simulink model "sol_mdl"  (R2024b)
settings: Solver=ode4  StartTime=0.0  StopTime=tf_sim  FixedStep=dt  RelTol=1e-3
values from neighbouring files (symbols this model uses):
  controller_coeffs = [Kp;Kd]    [init.m]
  q0_c1 = angle2quat(teta0_c1(3),teta0_c1(2),teta0_c1(1),'ZYX')    [init.m]
  q0_c2 = angle2quat(teta0_c2(3),teta0_c2(2),teta0_c2(1),'ZYX')    [init.m]
  qd_c1 = angle2quat(tetad_c1(3),tetad_c1(2),tetad_c1(1),'ZYX')    [init.m]
  qd_c2 = angle2quat(tetad_c2(3),tetad_c2(2),tetad_c2(1),'ZYX')    [init.m]
  so_c1 = Cbo'*sb0    [init.m]
  so_c2 = Cbo'*sb0    [init.m]
  system_parameters = [a; l; b; As; sigma; ms; mp; mr; mt; P]    [init.m]
  tetad_c2 = deg2rad([0 20 20]')    [init.m]
  w0_c1 = [0 5 5]'*1e-4    [init.m]
  w0_c2 = [0 0 0]'    [init.m]
libraries: aerolibutil x4, sharedtransform x2, simulink_extras x2
settings Model: Creator=Monster  LastModifiedBy=Monster

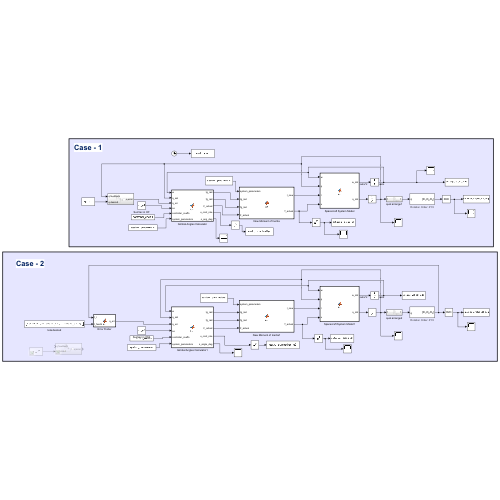
[thumbnail: Simulink's stored preview of the top-level diagram]
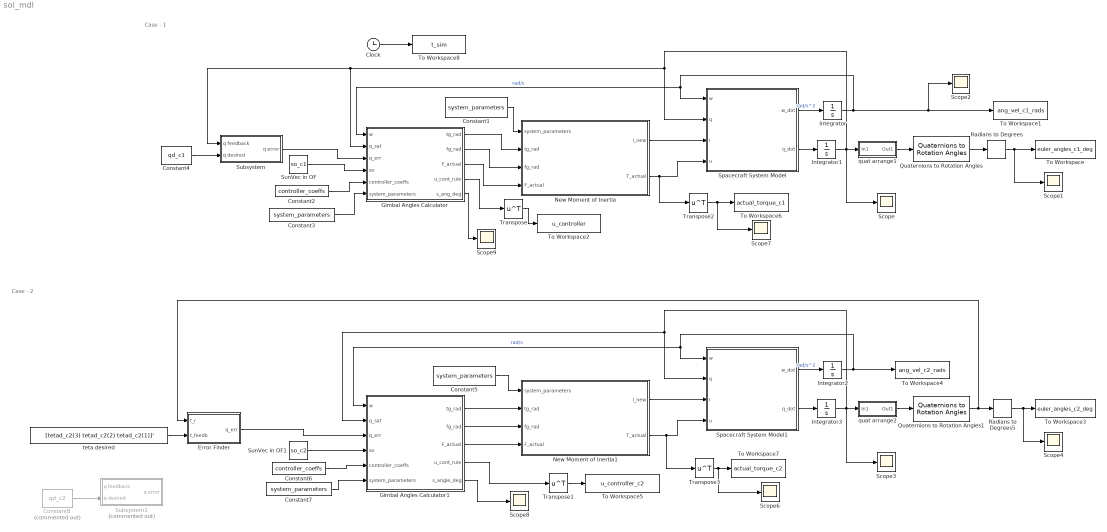
== system sol_mdl ==
  note: Case - 1
  note: Case - 2
  Clock : Clock
  Constant{1,3,5,7} (4 alike) : Constant  Value=system_parameters
  Constant2 : Constant  Value=controller_coeffs
  Constant4 : Constant  Value=qd_c1
  Constant6 : Constant  Value=controller_coeffs
  Constant8 : Constant  Commented=on  Value=qd_c2
  Error Finder : MATLAB Function  TreatAsAtomicUnit=on
  Gimbal Angles Calculator : MATLAB Function  TreatAsAtomicUnit=on
  Gimbal Angles Calculator1 : MATLAB Function  TreatAsAtomicUnit=on
  Integrator : Integrator  InitialCondition=w0_c1
  Integrator1 : Integrator  InitialCondition=[q0_c1(2:4)';q0_c1(1)]
  Integrator2 : Integrator  InitialCondition=w0_c2
  Integrator3 : Integrator  InitialCondition=[q0_c2(2:4)';q0_c2(1)]
  New Moment of Inertia : MATLAB Function  TreatAsAtomicUnit=on
  New Moment of Inertia1 : MATLAB Function  TreatAsAtomicUnit=on
  Quaternions to Rotation Angles : sharedtransform/Quaternions to Rotation Angles  rotationOrder=ZYX  aMode=aMode
  Quaternions to Rotation Angles1 : sharedtransform/Quaternions to Rotation Angles  rotationOrder=ZYX  aMode=aMode
  Radians to Degrees : simulink_extras/Transformations/Radians to Degrees
  Radians to Degrees5 : simulink_extras/Transformations/Radians to Degrees
  Scope{,1..4,6..9} (9 alike) : Scope
  Spacecraft System Model : MATLAB Function  TreatAsAtomicUnit=on
  Spacecraft System Model1 : MATLAB Function  TreatAsAtomicUnit=on
  Subsystem : Subsystem
  Subsystem1 : Subsystem  Commented=on
  SunVec in OF : Constant  Value=so_c1
  SunVec in OF1 : Constant  Value=so_c2
  To Workspace : ToWorkspace  VariableName=euler_angles_c1_deg  SampleTime=-1
      settings: Save2DSignal=2-D array (concatenate along first dimension)
  To Workspace1 : ToWorkspace  VariableName=ang_vel_c1_rads  SampleTime=-1
      settings: Save2DSignal=2-D array (concatenate along first dimension)
  To Workspace2 : ToWorkspace  VariableName=u_controller  SampleTime=-1
      settings: Save2DSignal=2-D array (concatenate along first dimension)
  To Workspace3 : ToWorkspace  VariableName=euler_angles_c2_deg  SampleTime=-1
      settings: Save2DSignal=2-D array (concatenate along first dimension)
  To Workspace4 : ToWorkspace  VariableName=ang_vel_c2_rads  SampleTime=-1
      settings: Save2DSignal=2-D array (concatenate along first dimension)
  To Workspace5 : ToWorkspace  VariableName=u_controller_c2  SampleTime=-1
      settings: Save2DSignal=2-D array (concatenate along first dimension)
  To Workspace6 : ToWorkspace  VariableName=actual_torque_c1  SampleTime=-1
      settings: Save2DSignal=2-D array (concatenate along first dimension)
  To Workspace7 : ToWorkspace  VariableName=actual_torque_c2  SampleTime=-1
      settings: Save2DSignal=2-D array (concatenate along first dimension)
  To Workspace8 : ToWorkspace  VariableName=t_sim  SampleTime=-1
      settings: Save2DSignal=2-D array (concatenate along first dimension)
  Transpose{,1..3} (4 alike) : Math  Operator=transpose
  quat arrange1 : Subsystem
  quat arrange2 : Subsystem
  teta desired : Constant  Value=[tetad_c2(3) tetad_c2(2) tetad_c2(1)]'
  wires:
  Spacecraft System Model/2(q_dot) -> Integrator1/1
  Spacecraft System Model/1(w_dot) -> Integrator/1  "rad/s^2"
  Integrator/1 -> Scope2/1, To Workspace1/1, Gimbal Angles Calculator/1(w), Spacecraft System Model/1(w)  "rad/s"
  Constant1/1 -> New Moment of Inertia/1(system_parameters)
  New Moment of Inertia/1(I_new) -> Spacecraft System Model/3(I)
  Quaternions to Rotation Angles/1 -> Radians to Degrees/1
  Constant2/1 -> Gimbal Angles Calculator/5(controller_coeffs)
  Gimbal Angles Calculator/1(tg_rad) -> New Moment of Inertia/2(tg_rad)
  Gimbal Angles Calculator/2(fg_rad) -> New Moment of Inertia/3(fg_rad)
  SunVec in OF/1 -> Gimbal Angles Calculator/4(so)
  Constant3/1 -> Gimbal Angles Calculator/6(system_parameters)
  Constant4/1 -> Subsystem/2(q desired)
  Subsystem/1(q error) -> Gimbal Angles Calculator/3(q_err)
  Gimbal Angles Calculator/3(F_actual) -> New Moment of Inertia/4(F_actual)
  New Moment of Inertia/2(T_actual) -> Transpose2/1, Spacecraft System Model/4(u)
  Gimbal Angles Calculator/4(u_cont_rule) -> Transpose/1
  Transpose/1 -> To Workspace2/1
  Radians to Degrees/1 -> Scope1/1, To Workspace/1
  Integrator1/1 -> Scope/1, Gimbal Angles Calculator/2(q_sat), Subsystem/1(q feedback), Spacecraft System Model/2(q), quat arrange1/1(In1)
  quat arrange1/1(Out1) -> Quaternions to Rotation Angles/1
  quat arrange2/1(Out1) -> Quaternions to Rotation Angles1/1
  Integrator3/1 -> quat arrange2/1(In1), Spacecraft System Model1/2(q), Gimbal Angles Calculator1/2(q_sat), Scope3/1
  Quaternions to Rotation Angles1/1 -> Error Finder/1(t_r), Radians to Degrees5/1
  Transpose1/1 -> To Workspace5/1
  Gimbal Angles Calculator1/4(u_cont_rule) -> Transpose1/1
  Gimbal Angles Calculator1/3(F_actual) -> New Moment of Inertia1/4(F_actual)
  Constant8/1 -> Subsystem1/2(q desired)
  Constant7/1 -> Gimbal Angles Calculator1/6(system_parameters)
  SunVec in OF1/1 -> Gimbal Angles Calculator1/4(so)
  Gimbal Angles Calculator1/2(fg_rad) -> New Moment of Inertia1/3(fg_rad)
  Gimbal Angles Calculator1/1(tg_rad) -> New Moment of Inertia1/2(tg_rad)
  Constant6/1 -> Gimbal Angles Calculator1/5(controller_coeffs)
  New Moment of Inertia1/1(I_new) -> Spacecraft System Model1/3(I)
  Constant5/1 -> New Moment of Inertia1/1(system_parameters)
  Integrator2/1 -> Spacecraft System Model1/1(w), Gimbal Angles Calculator1/1(w), To Workspace4/1  "rad/s"
  Spacecraft System Model1/1(w_dot) -> Integrator2/1  "rad/s^2"
  Spacecraft System Model1/2(q_dot) -> Integrator3/1
  Transpose2/1 -> Scope7/1, To Workspace6/1
  Transpose3/1 -> Scope6/1, To Workspace7/1
  New Moment of Inertia1/2(T_actual) -> Transpose3/1, Spacecraft System Model1/4(u)
  Gimbal Angles Calculator1/5(s_angle_deg) -> Scope8/1
  Gimbal Angles Calculator/5(s_ang_deg) -> Scope9/1
  teta desired/1 -> Error Finder/2(t_feedb)
  Radians to Degrees5/1 -> To Workspace3/1, Scope4/1
  Error Finder/1(q_err) -> Gimbal Angles Calculator1/3(q_err)
  Clock/1 -> To Workspace8/1

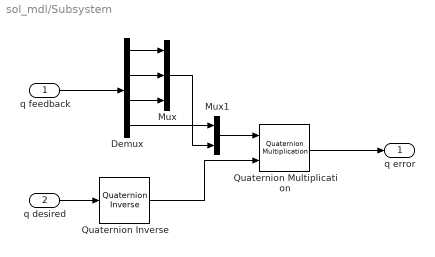
== system sol_mdl/Subsystem ==
  q feedback : Inport
  q desired : Inport  Port=2
  Demux : Demux
  Mux : Mux  Inputs=3
  Mux1 : Mux  Inputs=2
  Quaternion Inverse : aerolibutil/Quaternion Inverse
  Quaternion Multiplication : aerolibutil/Quaternion Multiplication
  q error : Outport
  wires:
  q desired/1 -> Quaternion Inverse/1
  Quaternion Inverse/1 -> Quaternion Multiplication/2
  q feedback/1 -> Demux/1
  Quaternion Multiplication/1 -> q error/1
  Mux/1 -> Mux1/2
  Mux1/1 -> Quaternion Multiplication/1
  Demux/2 -> Mux/2
  Demux/1 -> Mux/1
  Demux/3 -> Mux/3
  Demux/4 -> Mux1/1

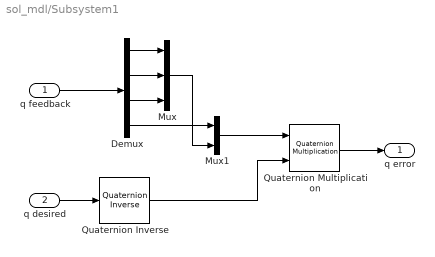
== system sol_mdl/Subsystem1 ==
  q feedback : Inport
  q desired : Inport  Port=2
  Demux : Demux
  Mux : Mux  Inputs=3
  Mux1 : Mux  Inputs=2
  Quaternion Inverse : aerolibutil/Quaternion Inverse
  Quaternion Multiplication : aerolibutil/Quaternion Multiplication
  q error : Outport
  wires:
  Demux/4 -> Mux1/1
  Demux/3 -> Mux/3
  Demux/1 -> Mux/1
  Demux/2 -> Mux/2
  Mux1/1 -> Quaternion Multiplication/1
  Mux/1 -> Mux1/2
  Quaternion Multiplication/1 -> q error/1
  q feedback/1 -> Demux/1
  Quaternion Inverse/1 -> Quaternion Multiplication/2
  q desired/1 -> Quaternion Inverse/1

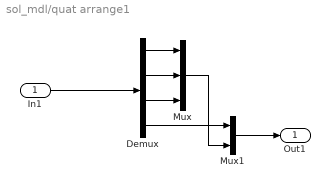
== system sol_mdl/quat arrange1 ==
  In1 : Inport
  Demux : Demux
  Mux : Mux  Inputs=3
  Mux1 : Mux  Inputs=2
  Out1 : Outport
  wires:
  Demux/4 -> Mux1/1
  Mux1/1 -> Out1/1
  Demux/1 -> Mux/1
  In1/1 -> Demux/1
  Demux/3 -> Mux/3
  Mux/1 -> Mux1/2
  Demux/2 -> Mux/2

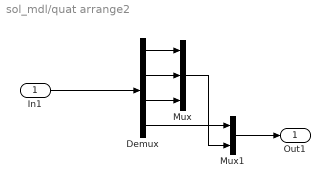
== system sol_mdl/quat arrange2 ==
  In1 : Inport
  Demux : Demux
  Mux : Mux  Inputs=3
  Mux1 : Mux  Inputs=2
  Out1 : Outport
  wires:
  Demux/2 -> Mux/2
  Mux/1 -> Mux1/2
  Demux/3 -> Mux/3
  In1/1 -> Demux/1
  Demux/1 -> Mux/1
  Mux1/1 -> Out1/1
  Demux/4 -> Mux1/1

== matlab function sol_mdl/Gimbal Angles Calculator1 ==
  data: w input; q_sat input; q_err input; so input; tg_rad output; fg_rad output; F_actual output; controller_coeffs input; u_cont_rule output; system_parameters input; s_angle_deg output
function [tg_rad,fg_rad,F_actual,u_cont_rule,s_angle_deg] = fcn(w,q_sat,q_err,so,controller_coeffs, system_parameters)

%% Arrange the quaternion
% q_sat_err = [q_err(2:4); q_err(1)];
q_sat_err = q_err;

%% Obtain the system parameters

a     = system_parameters(1);  % sail side length [meter]
l     = system_parameters(2);  % gimballed rod length [meter]
b     = system_parameters(3);  % Gimball Mechanism Height [meter]
As    = system_parameters(4);  % Sail Area [m^2]
sigma = system_parameters(5);  % Thrust Coefficient
ms    = system_parameters(6);  % Sail Subsystem Mass [kg]
mp    = system_parameters(7);  % Payload Mass [kg]
mr    = system_parameters(8);  % Gimballed Rod Mass [kg]
mt    = system_parameters(9);  % total mass [kg]
P     = system_parameters(10);


%% Applied PD Controller Rule
Kp = controller_coeffs(1);
Kd = controller_coeffs(2);

% Proportional Matrice
I3x3 = eye(3,3);
K = Kp*I3x3;
% Derivative Matrice
C = Kd*I3x3;

% Controller Output
u_cont_rule  = -K*q_sat_err(1:3) - C*w;

Tb1 = u_cont_rule(1);
Tb2 = u_cont_rule(2);
Tb3 = u_cont_rule(3);

%% Calculation of Gimbal Angles

eps = q_sat(1:3);
nu  = q_sat(4);
I3x3 = eye(3);

eps_cross_mat = crossMat(eps);
Cbo = (1-2*(eps')*eps)*I3x3 + 2*eps*eps' - 2*nu*eps_cross_mat;

sb = Cbo*so;

sb1 = sb(1); 

fg_rad = atan(Tb2/Tb3);
 
if fg_rad > pi/2
    fg_rad = pi/2;
elseif fg_rad < -pi/2
        fg_rad = -pi/2;
end

numt = Tb3*mt;
dent = sigma*P*As*(sb1^2)*l*cos(fg_rad)*(mp+mr/2);

tg_rad = asin(numt/dent);

if numt/dent > 1
    tg_rad = pi/2;
elseif numt/dent < -1
    tg_rad = -pi/2;
end

%% Actual Force Calculation
F_actual = sigma*P*As*(sb1^2);

%% Sun Angle Change
s_angle_deg = acosd(sb1);

end

== matlab function sol_mdl/New Moment of Inertia ==
  data: system_parameters input; I_new output; tg_rad input; fg_rad input; F_actual input; T_actual output
function [I_new,T_actual] = fcn(system_parameters, tg_rad, fg_rad, F_actual)

%% Obtain the system parameters
a     = system_parameters(1);  % sail side length [meter]
l     = system_parameters(2);  % gimballed rod length [meter]
b     = system_parameters(3);  % Gimball Mechanism Height [meter]
As    = system_parameters(4);  % Sail Area [m^2]
sigma = system_parameters(5);  % Thrust Coefficient
ms    = system_parameters(6);  % Sail Subsystem Mass [kg]
mp    = system_parameters(7);  % Payload Mass [kg]
mr    = system_parameters(8);  % Gimballed Rod Mass [kg]
mt    = system_parameters(9);  % total mass [kg]
P     = system_parameters(10);  % total mass [kg]

%% Calculation of Center of Masses
xc_p = b + l*cos(tg_rad);
yc_p = l*sin(tg_rad)*cos(fg_rad);
zc_p = l*sin(tg_rad)*sin(fg_rad);

Xp_cm = [xc_p yc_p zc_p]';

xc_r = 0.5*xc_p;
yc_r = 0.5*yc_p;
zc_r = 0.5*zc_p;

Xr_cm = [xc_r yc_r zc_r]';

Xs_cm = [0 0 0]';

xc_mt = (mp*xc_p + mr*xc_r)/mt;
yc_mt = (mp*yc_p + mr*yc_r)/mt;
zc_mt = (mp*zc_p + mr*zc_r)/mt;

X_cm = [xc_mt yc_mt zc_mt]';

%% Moment of Inertia of Components in the Components Frame
Is_C = (ms/12)*diag([2*a^2 a^2 a^2]);
Ir_C = (mr*l^2/12)*diag([0 1 1]);

% Rotation Matrice from sail frame to the spacecraft
ang_bs_b1 = deg2rad(45);
Cbs_b1 = [1              0               0; 
          0 cos(ang_bs_b1) -sin(ang_bs_b1);
          0 sin(ang_bs_b1)  cos(ang_bs_b1)];

% Moment of Inertia of Sail Subsystem in the Body Frame
Is_B = Cbs_b1*Is_C*(Cbs_b1');

% Rotation Matrice from the gimball frame to the spacecraft frame,
Cbg_b1 = [1              0               0; 
          0    cos(fg_rad)    -sin(fg_rad);
          0    sin(fg_rad)     cos(fg_rad)];
Cbg_b3 = [cos(-tg_rad) -sin(-tg_rad)  0;
          sin(-tg_rad)  cos(-tg_rad)  0;
                    1             0   0];

Cbg = Cbg_b1*Cbg_b3;

Ir_B = Cbg*Ir_C*(Cbg');

% Calculaton of New Inertial

dX_p = Xp_cm - X_cm;
dX_r = Xr_cm - X_cm;
dX_s = Xs_cm - X_cm;

I11_p = mp*(dX_p(2)^2 + dX_p(3)^2);
I11_r = Ir_B(1,1) + mr*(dX_r(2)^2 + dX_r(3)^2);
I11_s = Is_B(1,1) + ms*(dX_s(2)^2 + dX_s(3)^2);
I11 = I11_p + I11_r + I11_s;

I22_p = mp*(dX_p(1)^2 + dX_p(3)^2);
I22_r = Ir_B(2,2) + mr*(dX_r(1)^2 + dX_r(3)^2);
I22_s = Is_B(2,2) + ms*(dX_s(1)^2 + dX_s(3)^2);
I22 = I22_p + I22_r + I22_s;

I33_p = mp*(dX_p(1)^2 + dX_p(2)^2);
I33_r = Ir_B(3,3) + mr*(dX_r(1)^2 + dX_r(2)^2);
I33_s = Is_B(3,3) + ms*(dX_s(1)^2 + dX_s(2)^2);
I33 = I33_p + I33_r + I33_s;

I12_p = mp*dX_p(1)*dX_p(2);
I12_r = Ir_B(1,2) + mr*dX_r(1)*dX_r(2);
I12_s = Is_B(1,2) + ms*dX_s(1)*dX_s(2);
I12   = I12_p + I12_r + I12_s;
I21   = I12;

I23_p = mp*dX_p(2)*dX_p(3);
I23_r = Ir_B(2,3) + mr*dX_r(2)*dX_r(3);
I23_s = Is_B(2,3) + ms*dX_s(2)*dX_s(3);
I23   = I23_p + I23_r + I23_s;
I32   = I23;

I13_p = mp*dX_p(1)*dX_p(3);
I13_r = Ir_B(1,3) + mr*dX_r(1)*dX_r(3);
I13_s = Is_B(1,3) + ms*dX_s(1)*dX_s(3);
I13   = I13_p + I13_r + I13_s;
I31   = I13;

% Output
I_new = [I11 I12 I13
         I21 I22 I23
         I31 I32 I33];

%% Actual Control Torque Calculation

T_b1 = 0;
T_b2 = F_actual*zc_mt;
T_b3 = F_actual*yc_mt;

T_actual = [T_b1;T_b2;T_b3];

end

== matlab function sol_mdl/Gimbal Angles Calculator ==
  data: w input; q_sat input; q_err input; so input; tg_rad output; fg_rad output; F_actual output; controller_coeffs input; u_cont_rule output; system_parameters input; s_ang_deg output
function [tg_rad,fg_rad,F_actual,u_cont_rule,s_ang_deg] = fcn(w,q_sat,q_err,so,controller_coeffs, system_parameters)

%% Arrange the quaternion
q = [q_err(2:4); q_err(1)];

%% Obtain the system parameters

a     = system_parameters(1);  % sail side length [meter]
l     = system_parameters(2);  % gimballed rod length [meter]
b     = system_parameters(3);  % Gimball Mechanism Height [meter]
As    = system_parameters(4);  % Sail Area [m^2]
sigma = system_parameters(5);  % Thrust Coefficient
ms    = system_parameters(6);  % Sail Subsystem Mass [kg]
mp    = system_parameters(7);  % Payload Mass [kg]
mr    = system_parameters(8);  % Gimballed Rod Mass [kg]
mt    = system_parameters(9);  % total mass [kg]
P     = system_parameters(10);


%% Applied PD Controller Rule
Kp = controller_coeffs(1);
Kd = controller_coeffs(2);

% Proportional Matrice
I3x3 = eye(3,3);
K = Kp*I3x3;
% Derivative Matrice
C = Kd*I3x3;

% Controller Output
u_cont_rule  = -K*q(1:3) - C*w;

Tb1 = u_cont_rule(1);
Tb2 = u_cont_rule(2);
Tb3 = u_cont_rule(3);

%% Calculation of Gimbal Angles

eps = q_sat(1:3);
nu  = q_sat(4);
I3x3 = eye(3);

eps_cross_mat = crossMat(eps);
Cbo = (1-2*(eps')*eps)*I3x3 + 2*eps*eps' - 2*nu*eps_cross_mat;

sb = Cbo*so;

sb1 = sb(1); 

fg_rad = atan(Tb2/Tb3);
 
if fg_rad > pi/2
    fg_rad = pi/2;
elseif fg_rad < -pi/2
        fg_rad = -pi/2;
end

numt = Tb3*mt;
dent = sigma*P*As*(sb1^2)*l*cos(fg_rad)*(mp+mr/2);

tg_rad = asin(numt/dent);

if numt/dent > 1
    tg_rad = pi/2;
elseif numt/dent < -1
    tg_rad = -pi/2;
end

%% Actual Force Calculation
F_actual = sigma*P*As*(sb1^2);

%% Angle sun vector
s_ang_deg = acosd(sb1);

end

== matlab function sol_mdl/New Moment of Inertia1 ==
  data: system_parameters input; I_new output; tg_rad input; fg_rad input; F_actual input; T_actual output
function [I_new,T_actual] = fcn(system_parameters, tg_rad, fg_rad, F_actual)

%% Obtain the system parameters
a     = system_parameters(1);  % sail side length [meter]
l     = system_parameters(2);  % gimballed rod length [meter]
b     = system_parameters(3);  % Gimball Mechanism Height [meter]
As    = system_parameters(4);  % Sail Area [m^2]
sigma = system_parameters(5);  % Thrust Coefficient
ms    = system_parameters(6);  % Sail Subsystem Mass [kg]
mp    = system_parameters(7);  % Payload Mass [kg]
mr    = system_parameters(8);  % Gimballed Rod Mass [kg]
mt    = system_parameters(9);  % total mass [kg]
P     = system_parameters(10);  % total mass [kg]

%% Calculation of Center of Masses
xc_p = b + l*cos(tg_rad);
yc_p = l*sin(tg_rad)*cos(fg_rad);
zc_p = l*sin(tg_rad)*sin(fg_rad);

Xp_cm = [xc_p yc_p zc_p]';

xc_r = 0.5*xc_p;
yc_r = 0.5*yc_p;
zc_r = 0.5*zc_p;

Xr_cm = [xc_r yc_r zc_r]';

Xs_cm = [0 0 0]';

xc_mt = (mp*xc_p + mr*xc_r)/mt;
yc_mt = (mp*yc_p + mr*yc_r)/mt;
zc_mt = (mp*zc_p + mr*zc_r)/mt;

X_cm = [xc_mt yc_mt zc_mt]';

%% Moment of Inertia of Components in the Components Frame
Is_C = (ms/12)*diag([2*a^2 a^2 a^2]);
Ir_C = (mr*l^2/12)*diag([0 1 1]);

% Rotation Matrice from sail frame to the spacecraft
ang_bs_b1 = deg2rad(45);
Cbs_b1 = [1              0               0; 
          0 cos(ang_bs_b1) -sin(ang_bs_b1);
          0 sin(ang_bs_b1)  cos(ang_bs_b1)];

% Moment of Inertia of Sail Subsystem in the Body Frame
Is_B = Cbs_b1*Is_C*(Cbs_b1');

% Rotation Matrice from the gimball frame to the spacecraft frame,
Cbg_b1 = [1              0               0; 
          0    cos(fg_rad)    -sin(fg_rad);
          0    sin(fg_rad)     cos(fg_rad)];
Cbg_b3 = [cos(-tg_rad) -sin(-tg_rad)  0;
          sin(-tg_rad)  cos(-tg_rad)  0;
                    1             0   0];

Cbg = Cbg_b1*Cbg_b3;

Ir_B = Cbg*Ir_C*(Cbg');

% Calculaton of New Inertial

dX_p = Xp_cm - X_cm;
dX_r = Xr_cm - X_cm;
dX_s = Xs_cm - X_cm;

I11_p = mp*(dX_p(2)^2 + dX_p(3)^2);
I11_r = Ir_B(1,1) + mr*(dX_r(2)^2 + dX_r(3)^2);
I11_s = Is_B(1,1) + ms*(dX_s(2)^2 + dX_s(3)^2);
I11 = I11_p + I11_r + I11_s;

I22_p = mp*(dX_p(1)^2 + dX_p(3)^2);
I22_r = Ir_B(2,2) + mr*(dX_r(1)^2 + dX_r(3)^2);
I22_s = Is_B(2,2) + ms*(dX_s(1)^2 + dX_s(3)^2);
I22 = I22_p + I22_r + I22_s;

I33_p = mp*(dX_p(1)^2 + dX_p(2)^2);
I33_r = Ir_B(3,3) + mr*(dX_r(1)^2 + dX_r(2)^2);
I33_s = Is_B(3,3) + ms*(dX_s(1)^2 + dX_s(2)^2);
I33 = I33_p + I33_r + I33_s;

I12_p = mp*dX_p(1)*dX_p(2);
I12_r = Ir_B(1,2) + mr*dX_r(1)*dX_r(2);
I12_s = Is_B(1,2) + ms*dX_s(1)*dX_s(2);
I12   = I12_p + I12_r + I12_s;
I21   = I12;

I23_p = mp*dX_p(2)*dX_p(3);
I23_r = Ir_B(2,3) + mr*dX_r(2)*dX_r(3);
I23_s = Is_B(2,3) + ms*dX_s(2)*dX_s(3);
I23   = I23_p + I23_r + I23_s;
I32   = I23;

I13_p = mp*dX_p(1)*dX_p(3);
I13_r = Ir_B(1,3) + mr*dX_r(1)*dX_r(3);
I13_s = Is_B(1,3) + ms*dX_s(1)*dX_s(3);
I13   = I13_p + I13_r + I13_s;
I31   = I13;

% Output
I_new = [I11 I12 I13
         I21 I22 I23
         I31 I32 I33];

%% Actual Control Torque Calculation

T_b1 = 0;
T_b2 = F_actual*zc_mt;
T_b3 = F_actual*yc_mt;

T_actual = [T_b1;T_b2;T_b3];

end

== matlab function sol_mdl/Spacecraft System Model1 ==
  data: w input; q input; w_dot output; I input; u input; q_dot output
function [w_dot,q_dot] = fcn(w,q,I,u)

% Spacecraft Dynamic

w1 = w(1);
w2 = w(2);
w3 = w(3);

W = [ 0,  w3, -w2, w1;
    -w3,   0,  w1, w2;
     w2, -w1,   0, w3;
    -w1, -w2, -w3,  0 ];

% output
w_dot = inv(I)*(-cross(w,I*w)+u);

q_dot = 0.5*W*q;

end

== matlab function sol_mdl/Error Finder ==
  data: t_r input; q_err output; t_feedb input
function q_err = fcn(t_r,t_feedb)
    
t_err = t_r - t_feedb;

Q = ypr2dcm321(t_err(1),t_err(2),t_err(3),'rad');

q_err = q_from_dcm(Q);

end

== matlab function sol_mdl/Spacecraft System Model ==
  data: w input; q input; w_dot output; I input; u input; q_dot output
function [w_dot,q_dot] = fcn(w,q,I,u)

% Spacecraft Dynamic

w1 = w(1);
w2 = w(2);
w3 = w(3);

W = [ 0,  w3, -w2, w1;
    -w3,   0,  w1, w2;
     w2, -w1,   0, w3;
    -w1, -w2, -w3,  0 ];

% output
w_dot = inv(I)*(-cross(w,I*w)+u);

q_dot = 0.5*W*q;

end
